simulink model "F_V_G"  (R2013a)
settings: Solver=ode45  StartTime=0.0  StopTime=0.2  RelTol=1e-3
settings Model: Creator=MEHEDI HASSAN  LastModifiedBy=MEHEDI HASSAN
settings OptimizationCC: InlineParams=on
settings DebuggingCC: SolverPrmCheckMsg=none  ModelReferenceExtraNoncontSigs=none

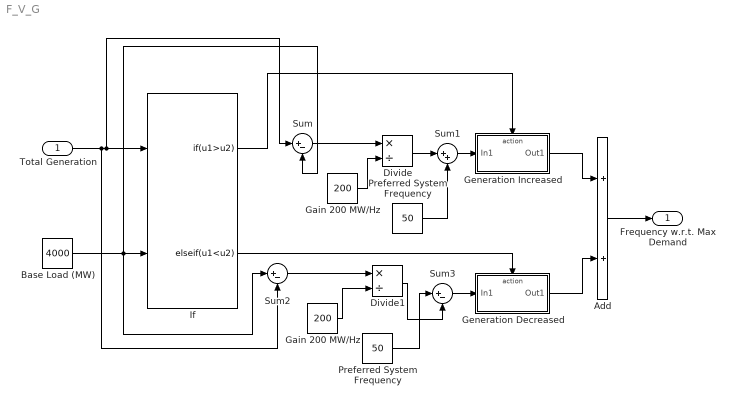
== system F_V_G ==
  Total Generation : Inport
  Add : Sum
  Base Load (MW) : Constant  Value=4000
  Divide : Product  Inputs=*/
  Divide1 : Product  Inputs=*/
  Gain 200 MW/Hz : Constant  Value=200
  "Gain 200 MW/Hz " : Constant  Value=200
  Generation Decreased : Subsystem  TreatAsAtomicUnit=on
  Generation Increased : Subsystem  TreatAsAtomicUnit=on
  If : If  NumInputs=2  IfExpression=u1>u2  ElseIfExpressions=u1<u2  ShowElse=off
  Preferred System Frequency : Constant  Value=50
  "Preferred System Frequency " : Constant  Value=50
  Sum : Sum  Inputs=|+-
  Sum1 : Sum  Inputs=|++
  Sum2 : Sum  Inputs=|+-
  Sum3 : Sum  Inputs=|+-
  Frequency w.r.t. Max Demand : Outport
  wires:
  Sum/1 -> Divide/1
  Gain 200 MW/Hz/1 -> Divide/2
  Divide/1 -> Sum1/1
  Preferred System Frequency/1 -> Sum1/2
  Sum1/1 -> Generation Increased/1(In1)
  Base Load (MW)/1 -> Sum/2, Sum2/1, If/2
  Sum2/1 -> Divide1/1
  "Gain 200 MW/Hz "/1 -> Divide1/2
  Divide1/1 -> Sum3/2
  "Preferred System Frequency "/1 -> Sum3/1
  Sum3/1 -> Generation Decreased/1(In1)
  Total Generation/1 -> Sum2/2, Sum/1, If/1
  If/1 -> Generation Increased/Action
  If/2 -> Generation Decreased/Action
  Generation Increased/1(Out1) -> Add/1
  Generation Decreased/1(Out1) -> Add/2
  Add/1 -> Frequency w.r.t. Max Demand/1

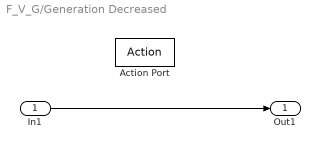
== system F_V_G/Generation Decreased ==
  In1 : Inport
  Action Port : ActionPort  ActionType=elseif
  Out1 : Outport
  wires:
  In1/1 -> Out1/1

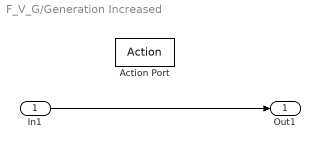
== system F_V_G/Generation Increased ==
  In1 : Inport
  Action Port : ActionPort  ActionType=then
  Out1 : Outport
  wires:
  In1/1 -> Out1/1
